simulink model "calculate_filter_coefficients"  (R2020b)
settings: Solver=FixedStepAuto  StartTime=0.0  StopTime=stopTime  RelTol=1e-3
libraries: FPGA_Open_Speech_Tools x2
settings Model: Creator=t96f346  LastModifiedBy=conno
settings DataIOCC: SaveOutput=off  SaveTime=off  ReturnWorkspaceOutputs=off
settings ModelReferenceCC: ModelReferenceNumInstancesAllowed=Single

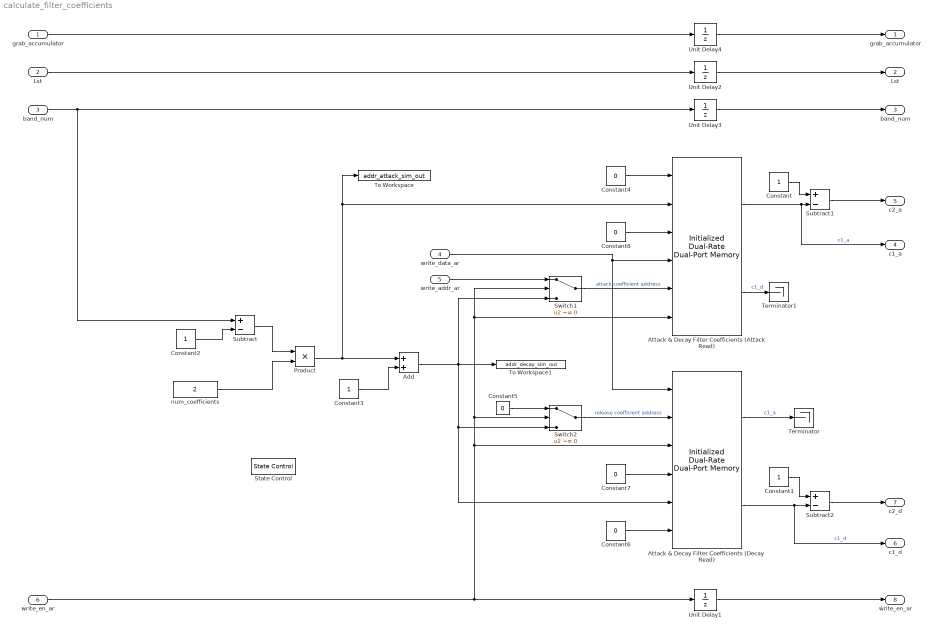
== system calculate_filter_coefficients ==
  grab_accumulator : Inport  OutDataTypeStr=boolean  PortDimensions=1
  Lst : Inport  Port=2  OutDataTypeStr=fixdt(1,40,32)  PortDimensions=1
  band_num : Inport  Port=3  OutDataTypeStr=uint8  PortDimensions=1
  write_data_ar : Inport  Port=4  OutDataTypeStr=fixdt(0,16,16)  PortDimensions=[1 1]
  write_addr_ar : Inport  Port=5  OutDataTypeStr=uint8  PortDimensions=[1 1]
  "write_en_ar " : Inport  Port=6  OutDataTypeStr=boolean  PortDimensions=[1 1]
  Add : Sum
  Attack & Decay Filter Coefficients (Attack Read) : FPGA_Open_Speech_Tools/Initialized Dual-Rate Dual-Port Memory  ram_size=coeff_size  Table_Init=ad_coeffs
      settings: SourceProductName=FPGA Open Speech Tools
  Attack & Decay Filter Coefficients (Decay Read) : FPGA_Open_Speech_Tools/Initialized Dual-Rate Dual-Port Memory  ram_size=coeff_size  Table_Init=ad_coeffs
      settings: SourceProductName=FPGA Open Speech Tools
  Constant{,1..3} (4 alike) : Constant  OutDataTypeStr=Inherit: Inherit via back propagation  SampleTime=-1
  Constant{4,6..8} (4 alike) : Constant  Value=0  OutDataTypeStr=Inherit: Inherit via back propagation  SampleTime=-1
  Constant5 : Constant  Value=0  OutDataTypeStr=uint8  SampleTime=-1
  Product : Product  OutDataTypeStr=uint8
  State Control : StateControl  StateControl=Synchronous
  Subtract : Sum  Inputs=+-
  Subtract1 : Sum  Inputs=+-  OutDataTypeStr=fixdt(0,16,16)
  Subtract2 : Sum  Inputs=+-  OutDataTypeStr=fixdt(0,16,16)
  Switch1 : Switch  Criteria=u2 ~= 0  OutDataTypeStr=Inherit: Inherit via back propagation
  Switch2 : Switch  Criteria=u2 ~= 0  OutDataTypeStr=uint8
  Terminator : Terminator
  Terminator1 : Terminator
  To Workspace : ToWorkspace  VariableName=addr_attack_sim_out  SampleTime=-1
  To Workspace1 : ToWorkspace  VariableName=addr_decay_sim_out  SampleTime=-1
  Unit Delay1 : UnitDelay  SampleTime=-1  HasFrameUpgradeWarning=on
  Unit Delay2 : UnitDelay  InitialCondition=65  SampleTime=-1  HasFrameUpgradeWarning=on
  Unit Delay3 : UnitDelay  InitialCondition=1  SampleTime=-1  HasFrameUpgradeWarning=on
  Unit Delay4 : UnitDelay  SampleTime=-1  HasFrameUpgradeWarning=on
  num_coefficients : Constant  Value=2  OutDataTypeStr=Inherit: Inherit via back propagation  SampleTime=-1
  "grab_accumulator " : Outport  PortDimensions=1
  "Lst " : Outport  Port=2  PortDimensions=1
  "band_num " : Outport  Port=3  PortDimensions=1
  c1_a : Outport  Port=4  PortDimensions=1
  c2_a : Outport  Port=5  PortDimensions=1
  c1_d : Outport  Port=6  PortDimensions=1
  c2_d : Outport  Port=7  PortDimensions=1
  write_en_ar : Outport  Port=8  PortDimensions=[1 1]
  wires:
  Attack & Decay Filter Coefficients (Attack Read)/2 -> Terminator1/1  "c1_d"
  Attack & Decay Filter Coefficients (Decay Read)/1 -> Terminator/1  "c1_a"
  Subtract1/1 -> c2_a/1
  Constant/1 -> Subtract1/1
  Attack & Decay Filter Coefficients (Attack Read)/1 -> c1_a/1, Subtract1/2  "c1_a"
  Constant4/1 -> Attack & Decay Filter Coefficients (Attack Read)/1
  Constant8/1 -> Attack & Decay Filter Coefficients (Attack Read)/3
  Unit Delay4/1 -> "grab_accumulator "/1
  grab_accumulator/1 -> Unit Delay4/1
  write_data_ar/1 -> Attack & Decay Filter Coefficients (Decay Read)/1, Attack & Decay Filter Coefficients (Attack Read)/4
  write_addr_ar/1 -> Switch1/1
  Subtract2/1 -> c2_d/1
  Unit Delay3/1 -> "band_num "/1
  Switch2/1 -> Attack & Decay Filter Coefficients (Decay Read)/2  "release coefficient address"
  Switch1/1 -> Attack & Decay Filter Coefficients (Attack Read)/5  "attack coefficient address"
  Lst/1 -> Unit Delay2/1
  Constant6/1 -> Attack & Decay Filter Coefficients (Decay Read)/6
  Constant7/1 -> Attack & Decay Filter Coefficients (Decay Read)/4
  Unit Delay1/1 -> write_en_ar/1
  Constant5/1 -> Switch2/1
  Unit Delay2/1 -> "Lst "/1
  Constant1/1 -> Subtract2/1
  Constant2/1 -> Subtract/2
  Attack & Decay Filter Coefficients (Decay Read)/2 -> Subtract2/2, c1_d/1  "c1_d"
  Constant3/1 -> Add/2
  Subtract/1 -> Product/1
  "write_en_ar "/1 -> Attack & Decay Filter Coefficients (Attack Read)/6, Switch1/2, Switch2/2, Attack & Decay Filter Coefficients (Decay Read)/3, Unit Delay1/1
  band_num/1 -> Subtract/1, Unit Delay3/1
  num_coefficients/1 -> Product/2
  Product/1 -> Attack & Decay Filter Coefficients (Attack Read)/2, To Workspace/1, Add/1
  Add/1 -> To Workspace1/1, Switch1/3, Attack & Decay Filter Coefficients (Decay Read)/5, Switch2/3
